simulink model "LQRRIP"  (Simulink 8.1)
settings: Solver=ode45  StartTime=0.0  StopTime=50  RelTol=1e-3
values from neighbouring files (symbols this model uses):
  K = lqr(A,B,Q,R)    [RIP.m]
settings Model: Creator=ThanhNhan  LastModifiedBy=ThanhNhan
settings DataIOCC: SignalLoggingSaveFormat=Dataset
settings OptimizationCC: ExpressionDepthLimit=128
settings DebuggingCC: FcnCallInpInsideContextMsg=EnableAllAsError
settings GRTTargetCC: CombineOutputUpdateFcns=on  GRTInterface=off

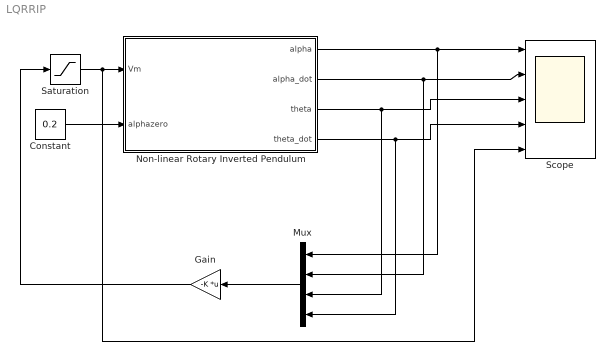
== system LQRRIP ==
  Constant : Constant  Value=0.2
  Gain : Gain  Gain=-K  Multiplication=Matrix(K*u)
  Mux : Mux
  Non-linear Rotary Inverted Pendulum : Subsystem  mask{Jeq=0.0148, g=9.81, m=0.05562, L=0.1254, r=0.1095, Beq=0.0444, eta=0.69, Km=0.084026, Kt=0.084039, Rm=2.6, Jm=0.001}
      mask prompts: Jeq "Momen quán tính tuong duong (Jeq)"; g "Gia toc trong truong (g)"; m "Khoi luong con lac (m)"; L "Nua chieu dai con lac (L)"; r "Nua chieu dài cánh tay (r)"; Beq "He so can tuong duong (Beq)"; eta "Hieu suat dong co (eta)"; Km "Hang so suc dien dong (Km)"; Kt "Hang so momen  (Kt)"; Rm "Dien tro phan ung (Rm)"; Jm "Momen quan tinh dong co (Jm)"
  Saturation : Saturate  UpperLimit=24  LowerLimit=-24
  Scope : Scope  NumInputPorts=5
      settings: TimeRange=0.1762452107279693  YMin=-0.1~-2~-2~-6~-28.52631578947364  YMax=0.3~1~0~2~-22.21052631578942
  wires:
  Constant/1 -> Non-linear Rotary Inverted Pendulum/2(alphazero)
  Mux/1 -> Gain/1
  Non-linear Rotary Inverted Pendulum/4(theta_dot) -> Scope/4, Mux/4
  Non-linear Rotary Inverted Pendulum/2(alpha_dot) -> Scope/2, Mux/2
  Non-linear Rotary Inverted Pendulum/1(alpha) -> Mux/1, Scope/1
  Gain/1 -> Saturation/1
  Saturation/1 -> Scope/5, Non-linear Rotary Inverted Pendulum/1(Vm)
  Non-linear Rotary Inverted Pendulum/3(theta) -> Mux/3, Scope/3

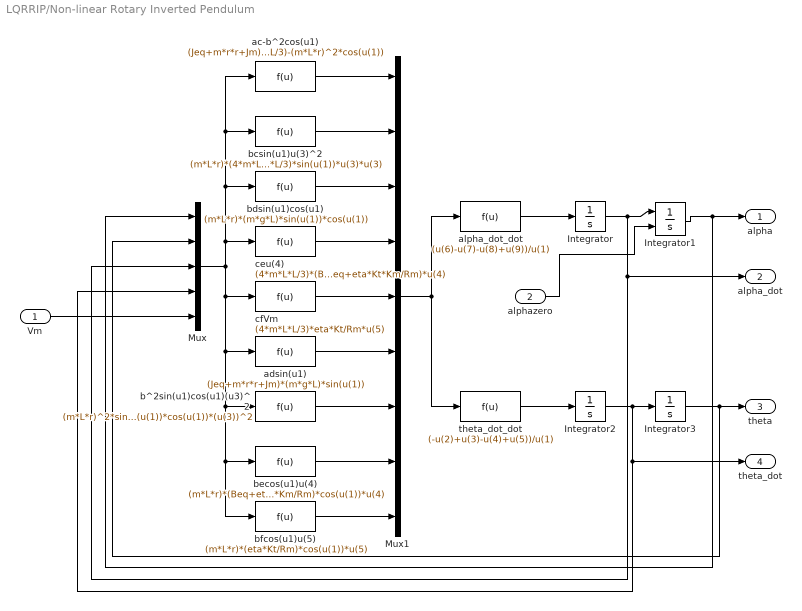
== system LQRRIP/Non-linear Rotary Inverted Pendulum ==
  Vm : Inport
  alphazero : Inport  Port=2
  Integrator : Integrator  UpperSaturationLimit=pi/18  LowerSaturationLimit=-pi/18
  Integrator1 : Integrator  InitialConditionSource=external  UpperSaturationLimit=pi/18  LowerSaturationLimit=-pi/18
  Integrator2 : Integrator
  Integrator3 : Integrator  UpperSaturationLimit=2  LowerSaturationLimit=-2
  Mux : Mux  Inputs=5
  Mux1 : Mux  Inputs=9
  ac-b^2cos(u1) : Fcn  Expr=(Jeq+m*r*r+Jm)*(4*m*L*L/3)-(m*L*r)^2*cos(u(1))
  adsin(u1) : Fcn  Expr=(Jeq+m*r*r+Jm)*(m*g*L)*sin(u(1))
  alpha_dot_dot : Fcn  Expr=(u(6)-u(7)-u(8)+u(9))/u(1)
  b^2sin(u1)cos(u1)(u3)^2 : Fcn  Expr=(m*L*r)^2*sin(u(1))*cos(u(1))*(u(3))^2
  bcsin(u1)u(3)^2 : Fcn  Expr=(m*L*r)*(4*m*L*L/3)*sin(u(1))*u(3)*u(3)
  bdsin(u1)cos(u1) : Fcn  Expr=(m*L*r)*(m*g*L)*sin(u(1))*cos(u(1))
  becos(u1)u(4) : Fcn  Expr=(m*L*r)*(Beq+eta*Kt*Km/Rm)*cos(u(1))*u(4)
  bfcos(u1)u(5) : Fcn  Expr=(m*L*r)*(eta*Kt/Rm)*cos(u(1))*u(5)
  ceu(4) : Fcn  Expr=(4*m*L*L/3)*(Beq+eta*Kt*Km/Rm)*u(4)
  cfVm : Fcn  Expr=(4*m*L*L/3)*eta*Kt/Rm*u(5)
  theta_dot_dot : Fcn  Expr=(-u(2)+u(3)-u(4)+u(5))/u(1)
  alpha : Outport
  alpha_dot : Outport  Port=2
  theta : Outport  Port=3
  theta_dot : Outport  Port=4
  wires:
  alpha_dot_dot/1 -> Integrator/1
  Integrator/1 -> Mux/3, alpha_dot/1, Integrator1/1
  theta_dot_dot/1 -> Integrator2/1
  Integrator1/1 -> Mux/1, alpha/1
  Integrator3/1 -> Mux/2, theta/1
  ac-b^2cos(u1)/1 -> Mux1/1
  bcsin(u1)u(3)^2/1 -> Mux1/2
  bdsin(u1)cos(u1)/1 -> Mux1/3
  ceu(4)/1 -> Mux1/4
  cfVm/1 -> Mux1/5
  adsin(u1)/1 -> Mux1/6
  b^2sin(u1)cos(u1)(u3)^2/1 -> Mux1/7
  becos(u1)u(4)/1 -> Mux1/8
  bfcos(u1)u(5)/1 -> Mux1/9
  Mux1/1 -> theta_dot_dot/1, alpha_dot_dot/1
  Mux/1 -> ceu(4)/1, bdsin(u1)cos(u1)/1, bcsin(u1)u(3)^2/1, ac-b^2cos(u1)/1, bfcos(u1)u(5)/1, becos(u1)u(4)/1, b^2sin(u1)cos(u1)(u3)^2/1, adsin(u1)/1, cfVm/1
  Integrator2/1 -> Mux/4, theta_dot/1, Integrator3/1
  Vm/1 -> Mux/5
  alphazero/1 -> Integrator1/2
